simulink model "lb533_usrp_tx_am_ssb"  (R2018b)
settings: Solver=VariableStepAuto  StartTime=0.0  StopTime=inf  RelTol=1e-3
undefined symbols (not defined in the file or in its folder): fdesignblkfcn, gcbh
libraries: dspsrcs4 x2, dspmlti4 x2, dspvision x1, dspfdesign x1, commsdrhw_v2 x1
settings Model: SimulationMode=accelerator  Creator=Григорий Фокин  LastModifiedBy=Григорий Фокин
settings SFSimCC: SimUseLocalCustomCode=off
settings RTWCC: RTWUseLocalCustomCode=off
settings CodeAppCC: StateflowObjectComments=on

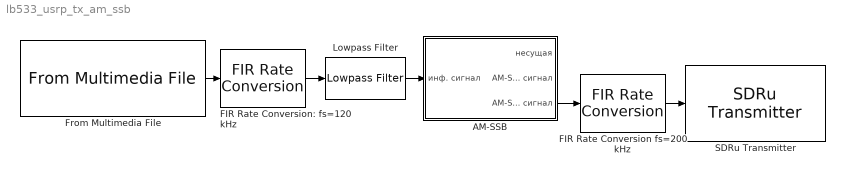
== system lb533_usrp_tx_am_ssb ==
  " AM-SSB" : Subsystem  mask{ac=2, ph=0, fc=40e3, fs=120e3, frame_size=1500}
      mask prompts: ac "Амплитуда поднесущей"; ph "Фаза поднесущей (рад)"; fc "Частота поднесущей (Гц)"; fs "Частота дискретизации (Гц)"; frame_size "Размер кадра (выборок)"
  FIR Rate Conversion fs=200 kHz : dspmlti4/FIR Rate Conversion  FilterSource=Dialog parameters  L=5  h=firpm(400, [0 55e3 65e3 600e3/2]/(600e3/2), [1 1 0 0], [1,1], 20)  M=3  FilterObject=FRC  roundingMode=Floor  overflowMode=off  firstCoeffDataTypeStr=Inherit: Same word length as input  firstCoeffMin=[]  firstCoeffMax=[]  firstCoeffLastDataTypeStr=Inherit: Same word length as input  outputDataTypeStr=Inherit: Same as accumulator  outputMin=[]  outputMax=[]  outputLastDataTypeStr=Inherit: Same as accumulator
      settings: SourceProductName=DSP System Toolbox  SourceProductBaseCode=DS
  FIR Rate Conversion: fs=120 kHz : dspmlti4/FIR Rate Conversion  FilterSource=Dialog parameters  L=5  h=firpm(50, [0 15e3 24e3 240e3/2]/(240e3/2), [1 1 0 0], [1,1], 20)  M=2  FilterObject=FRC  roundingMode=Floor  overflowMode=off  firstCoeffDataTypeStr=Inherit: Same word length as input  firstCoeffMin=[]  firstCoeffMax=[]  firstCoeffLastDataTypeStr=Inherit: Same word length as input  outputDataTypeStr=Inherit: Same as accumulator  outputMin=[]  outputMax=[]  outputLastDataTypeStr=Inherit: Same as accumulator
      settings: SourceProductName=DSP System Toolbox  SourceProductBaseCode=DS
  From Multimedia File : dspvision/From Multimedia File  inputFilename=C:\Users\Григорий Фокин\Documents\MATLAB\sut_study\dcsdr\audio_sources\music3_mono48kHz.wav  loop=on  numPlays=inf  outputStreams=Audio only  videoDataType=single  audioDataType=single  inheritSampleTime=on  userDefinedSampleTime=1/30  noAudioOutput=off  isIntensityVideo=off  fourcc=RGB  colorVideoFormat=Separate color signals  outputEOF=off  dataOrg=Column-major  audioFrameSize=600  computeAudioFrameSize=off  outSamplingMode=Sample based
      settings: SourceProductBaseCode=VP
  Lowpass Filter : dspfdesign/Lowpass Filter  FilterType=IIR  DesignForMinimumOrder=on  FilterOrder=20  PassbandFrequency=15e3  StopbandFrequency=16e3  PassbandRipple=0.01  StopbandAttenuation=80  InheritSampleRate=off  SampleRate=120e3  SimulateUsing=Interpreted execution  roundingMode=Floor  coeffsDataTypeStr=fixdt(1,16)
  SDRu Transmitter : commsdrhw_v2/SDRu Transmitter  rxtx=tx  initializeIPAddress=0  devMap=0  USRP2_IP=192.168.10.2  USRP_IP_X300=192.168.10.2  USRP_IP_X310=192.168.10.2  USRP_serialNumB200=No devices found  USRP_serialNumB210=F4E642  platform=B210  prevPlatform=B210  lastIPAddressPopup=192.168.10.2  USRP_ID=F4E642  LastIPAddress=192.168.10.2  ChannelMapping=1  centerFrequencySrc=Dialog  centerFrequency=1200e6  loOffsetSrc=Dialog  loOffset=0  gainSrc=Dialog  gain=70  PPSSource=Internal  clockSource=Internal  masterClkRateParam=6000000  masterClkRateB200=32e6  masterClkRateB210=6e6  masterClkRateX300=200e6  masterClkRateX310=200e6  decimInterpSrc=Dialog  decimInterp=30  USRP2_IP_NUM=[70 52 69 54 52 50]  frameLength=362  TransportDataType=int16  outputDatatype=Same as transport data type  overrunUnderrunPort=off  sampleTime=1  dboardInfo=|  HOST_DATA_PORT=30000  HOST_CONTROL_PORT=30001  USRP2_DATA_PORT=32769  USRP2_CONTROL_PORT=32768  bufferMode=Continuous streaming  EnableBurstMode=off  NumFramesInBurst=100
      | dbid: 0
      |           dbName: 'no db found'
      |          freqMin: 0
      |          freqMax: 0
      |          gainMin: 0
      |          gainMax: 0
      |     gainStepSize: 0
      settings: SourceProductName=Communications System Toolbox Support Package for USRP(R) Radio  SourceProductBaseCode=USRP
  wires:
  From Multimedia File/1 -> FIR Rate Conversion: fs=120 kHz/1
  FIR Rate Conversion: fs=120 kHz/1 -> Lowpass Filter/1
  FIR Rate Conversion fs=200 kHz/1 -> SDRu Transmitter/1
  Lowpass Filter/1 -> " AM-SSB"/1(инф. сигнал)
  " AM-SSB"/3(AM-SUSB сигнал) -> FIR Rate Conversion fs=200 kHz/1

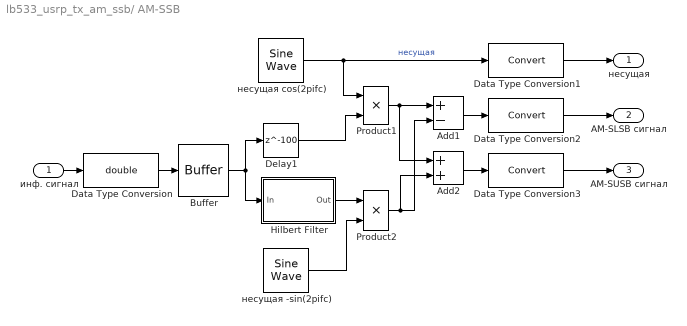
== system lb533_usrp_tx_am_ssb/ AM-SSB ==
  инф. сигнал : Inport
  Add1 : Sum  Inputs=+-
  Add2 : Sum
  Buffer : Buffer  N=frame_size  OutputFrames=off
  Data Type Conversion : DataTypeConversion  OutDataTypeStr=double
  Data Type Conversion1 : DataTypeConversion
  Data Type Conversion2 : DataTypeConversion
  Data Type Conversion3 : DataTypeConversion
  Delay1 : Delay  DelayLength=100  InitialCondition=0  InputProcessing=Columns as channels (frame based)
  Hilbert Filter : Subsystem  DialogController=fdesignblkfcn  InitFcn=fdesignblkfcn(gcbh, {'InitFcn'});  mask(Hilbert Filter){}
      mask help: Design a Hilbert filter
      settings: CopyFcn=fdesignblkfcn(gcbh, {'CopyFcn'});
      mask Help: helpview(mapfilelocation('dsp'), 'dsphilbertfilter');
      mask Display: disp('Hilbert')
  Product1 : Product
  Product2 : Product
  несущая cos(2pifc) : dspsrcs4/Sine Wave  Amplitude=ac  Frequency=fc  Phase=ph  SampleMode=Discrete  OutComplex=Real  CompMethod=Trigonometric fcn  TableSize=Speed  SampleTime=1/fs  SamplesPerFrame=frame_size  ResetState=Restart at time zero  OutputFrames=off  dataType=double  wordLen=16  udDataType=sfix(16)  fracBitsMode=Best precision  numFracBits=15  OutDataTypeStr=double  LastOutDataTypeStr=double
  несущая -sin(2pifc) : dspsrcs4/Sine Wave  Amplitude=ac  Frequency=fc  Phase=ph+(pi/2)  SampleMode=Discrete  OutComplex=Real  CompMethod=Trigonometric fcn  TableSize=Speed  SampleTime=1/fs  SamplesPerFrame=frame_size  ResetState=Restart at time zero  OutputFrames=off  dataType=double  wordLen=16  udDataType=sfix(16)  fracBitsMode=Best precision  numFracBits=15  OutDataTypeStr=double  LastOutDataTypeStr=double
  несущая : Outport
  AM-SLSB сигнал : Outport  Port=2
  AM-SUSB сигнал : Outport  Port=3
  wires:
  Buffer/1 -> Hilbert Filter/1(In), Delay1/1
  Data Type Conversion1/1 -> несущая/1
  Add2/1 -> Data Type Conversion3/1
  Delay1/1 -> Product1/2
  Product1/1 -> Add1/1, Add2/1
  инф. сигнал/1 -> Data Type Conversion/1
  Data Type Conversion3/1 -> AM-SUSB сигнал/1
  несущая cos(2pifc)/1 -> Data Type Conversion1/1, Product1/1  "несущая"
  Data Type Conversion2/1 -> AM-SLSB сигнал/1
  Hilbert Filter/1(Out) -> Product2/1
  Data Type Conversion/1 -> Buffer/1
  Add1/1 -> Data Type Conversion2/1
  Product2/1 -> Add2/2, Add1/2
  несущая -sin(2pifc)/1 -> Product2/2

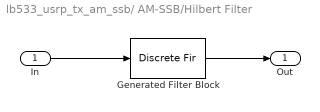
== system lb533_usrp_tx_am_ssb/ AM-SSB/Hilbert Filter ==
  In : Inport
  Generated Filter Block : DiscreteFir  Tag=BlockMethodSubSystem  Coefficients=[4.6653290912134353e-16 -8.3766156093727947e-05 2.3287802582575801e-15 -6.5992112024168155e-05 -6.2242128018656376e-16 -9.1525954819809117e-05 -1.9677454970641158e-15 -0.00012313243456045384 -4.0806315018380616e-16 -0.00016173066502496637 1.2958052328058529e-16 -0.00020842367058682403 1.9678295181986041e-15 -0.00026438321164375523 -1.7328150234907503e-15 -0.00033071001178729652 3.1411949301283626e-16 -0.00040869601103548205 3.2037105407109728e-16 -0.00049993156563202506 -1.144396980186295e-16 -0.00060563845625788513 -1.9855013969377896e-15 -0.00072769210664986976 2.3301185176846352e-16 -0.0008676799812968386 -1.0660682509940412e-15 -0.0010274756073032267 -1.6592993604014616e-16 -0.0012090153762093665 -1.3500585780807668e-15 -0.0014144071824740978 -3.8097754484021837e-17 -0.0016458472143358951 -1.3609392841277538e-15 -0.0019057282119867916 -2.5723640857395491e-16 -0.0021966459456658483 -2.8724410095925932e-15 -0.0025212720850087619 -3.3869531043604269e-16 -0.0028826317064054169 -2.5574919442074095e-15 -0.0032838882137394831 3.9171476907439256e-16 -0.0037285693279528048 -2.5357563526214699e-15 -0.0042205296067457237 -3.1399192896406897e-15 -0.0047640841311788473 -7.6967858620815603e-16 -0.0053640296699853096 -1.728112515457122e-15 -0.0060258227885992832 -2.3179779092842344e-15 -0.0067557074223738856 -1.96300714463523e-15 -0.007560867990307335 -3.8247083560239715e-15 -0.0084497865145100048 -8.0803541645689322e-16 -0.0094324724012080918 -2.017095154419686e-15 -0.010521000368820532 -3.3269892877592195e-15 -0.011730053960379405 -2.7272467188272053e-15 -0.013077802492927948 -1.3934035093686796e-15 -0.014586997591744755 -2.4123429358509422e-15 -0.01628665489541703 -2.1271681796355855e-15 -0.018214384178150911 -1.9674329921454366e-15 -0.020419872962853858 -2.0927949404138669e-15 -0.022970237720181919 -2.2092609555005438e-15 -0.025958314811609151 -2.0764457275676042e-15 -0.029516323722935001 -5.0279529284491431e-16 -0.033839039656023973 -2.9209256404834951e-15 -0.039225629524304084 -5.6888615390368565e-16 -0.046159968354213543 -1.965471466301946e-15 -0.055478713185773021 -2.2949631205154338e-16 -0.068763327967983567 -1.3355122304834698e-15 -0.089404236724446751 -6.5082869337524217e-16 -0.126218882474189 -5.2749556687355491e-16 -0.21154192368720315 -2.7459424026842848e-16 -0.63639794778019221 0 0.63639794778019221 2.7459424026842848e-16 0.21154192368720315 5.2749556687355491e-16 0.126218882474189 6.5082869337524217e-16 0.089404236724446751 1.3355122304834698e-15 0.068763327967983567 2.2949631205154338e-16 0.055478713185773021 1.965471466301946e-15 0.046159968354213543 5.6888615390368565e-16 0.039225629524304084 2.9209256404834951e-15 0.033839039656023973 5.0279529284491431e-16 0.029516323722935001 2.0764457275676042e-15 0.025958314811609151 2.2092609555005438e-15 0.022970237720181919 2.0927949404138669e-15 0.020419872962853858 1.9674329921454366e-15 0.018214384178150911 2.1271681796355855e-15 0.01628665489541703 2.4123429358509422e-15 0.014586997591744755 1.3934035093686796e-15 0.013077802492927948 2.7272467188272053e-15 0.011730053960379405 3.3269892877592195e-15 0.010521000368820532 2.017095154419686e-15 0.0094324724012080918 8.0803541645689322e-16 0.0084497865145100048 3.8247083560239715e-15 0.007560867990307335 1.96300714463523e-15 0.0067557074223738856 2.3179779092842344e-15 0.0060258227885992832 1.728112515457122e-15 0.0053640296699853096 7.6967858620815603e-16 0.0047640841311788473 3.1399192896406897e-15 0.0042205296067457237 2.5357563526214699e-15 0.0037285693279528048 -3.9171476907439256e-16 0.0032838882137394831 2.5574919442074095e-15 0.0028826317064054169 3.3869531043604269e-16 0.0025212720850087619 2.8724410095925932e-15 0.0021966459456658483 2.5723640857395491e-16 0.0019057282119867916 1.3609392841277538e-15 0.0016458472143358951 3.8097754484021837e-17 0.0014144071824740978 1.3500585780807668e-15 0.0012090153762093665 1.6592993604014616e-16 0.0010274756073032267 1.0660682509940412e-15 0.0008676799812968386 ...(+581 chars)]  InputProcessing=Columns as channels (frame based)
  Out : Outport
  wires:
  In/1 -> Generated Filter Block/1
  Generated Filter Block/1 -> Out/1
